simulink model "baxter_hybridcontroltraj2"  (Simulink 8.6)
settings: Solver=ode1  SolverMode=SingleTasking  StartTime=0.0  StopTime=stoptime  FixedStep=dt  RelTol=1e-3
values from neighbouring files (symbols this model uses):
  Aaug = [Ahat, zeros(14,7);Cpl(1:7,1:14), zeros(7)]    [mainMCVIntegralHybrid2_2d.m]
  Aaug1 = [Ahat1, zeros(14,7);Cpr(1:7,1:14), zeros(7)]    [mainMCVIntegralHybrid2_2d.m]
  Baug = [Bpl*Nbar Fhat; eye(7), zeros(7)]    [mainMCVIntegralHybrid2_2d.m]
  Baug1 = [Bpr*Nbar1 Fhat1; eye(7), zeros(7)]    [mainMCVIntegralHybrid2_2d.m]
  Caug = [eye(14),zeros(14,7)]    [mainMCVIntegralHybrid2_2d.m]
  Caug1 = [eye(14),zeros(14,7)]    [mainMCVIntegralHybrid2_2d.m]
  Daug = zeros(14,14)    [mainMCVIntegralHybrid2_2d.m]
  Daug1 = zeros(14,14)    [mainMCVIntegralHybrid2_2d.m]
  dt = 0.001    [mainMCVIntegralHybrid2_2d.m]
  faulttime = stoptime    (= 1795)    [mainMCVIntegralHybrid2_2d.m]
  initleft = [jlanglerow1(:,1)'+ 0.1*ones(1,7), zeros(1,14)]    [mainMCVIntegralHybrid2_2d.m]
  initright = [jranglerow1(:,1)'+ 0.1*ones(1,7),zeros(1,14)]    [mainMCVIntegralHybrid2_2d.m]
  Khat = Kplmcv    [mainMCVIntegralHybrid2_2d.m]
  seed = 0    [mainMCVIntegralHybrid2_2d.m]
  stepinput = [-0.36816     -0.55722      -1.1969       1.5731      0.99057       1.2609      0.60746].'    [mainMCVIntegralHybrid2_2d.m]
  stepinput1 = zeros(7,1)    [mainMCVIntegralHybrid2_2d.m]
  stepinput2 = [-0.36816     -0.55722      -1.1969       1.5731      0.99057       1.2609      0.60746].'    [mainMCVIntegralHybrid2_2d.m]
  steptime = 0.0    (= 0)    [mainMCVIntegralHybrid2_2d.m]
undefined symbols (not defined in the file or in its folder): jlanglerow, jranglerow, tanglerow
undefined symbols (not defined in the file): W
libraries: roblocks x14, powerlib_meascontrol x14
settings Model: Creator=Firdous  LastModifiedBy=Firdous
settings DataIOCC: LimitDataPoints=off  SaveFormat=Dataset  SignalLoggingSaveFormat=Dataset  ReturnWorkspaceOutputs=on
settings OptimizationCC: ExpressionDepthLimit=128
settings DebuggingCC: UnderspecifiedInitializationDetection=Simplified  MergeDetectMultiDrivingBlocksExec=error  SolverPrmCheckMsg=none  FcnCallInpInsideContextMsg=EnableAllAsError  AllowSymbolicDim=on  StateNameClashWarn=none  SFUnexpectedBacktrackingDiag=error  SFNoUnconditionalDefaultTransitionDiag=error
settings HardwareCC: ProdBitPerPointer=64  ProdLargestAtomicFloat=Float  ProdIntDivRoundTo=Zero  ProdEndianess=LittleEndian  ProdWordSize=64  ProdHWDeviceType=Intel->x86-64 (Windows64)
settings ModelReferenceCC: PropagateSignalLabelsOutOfModel=on
settings GRTTargetCC: TargetLangStandard=C99 (ISO)  GeneratePreprocessorConditionals=Use local settings  CombineOutputUpdateFcns=on  GRTInterface=off
settings ConfigComp: CovMetricSettings=dwe  CovHtmlReporting=off  CovSaveCumulativeToWorkspaceVar=off  CovSaveSingleToWorkspaceVar=off  CovExternalEMLEnable=on

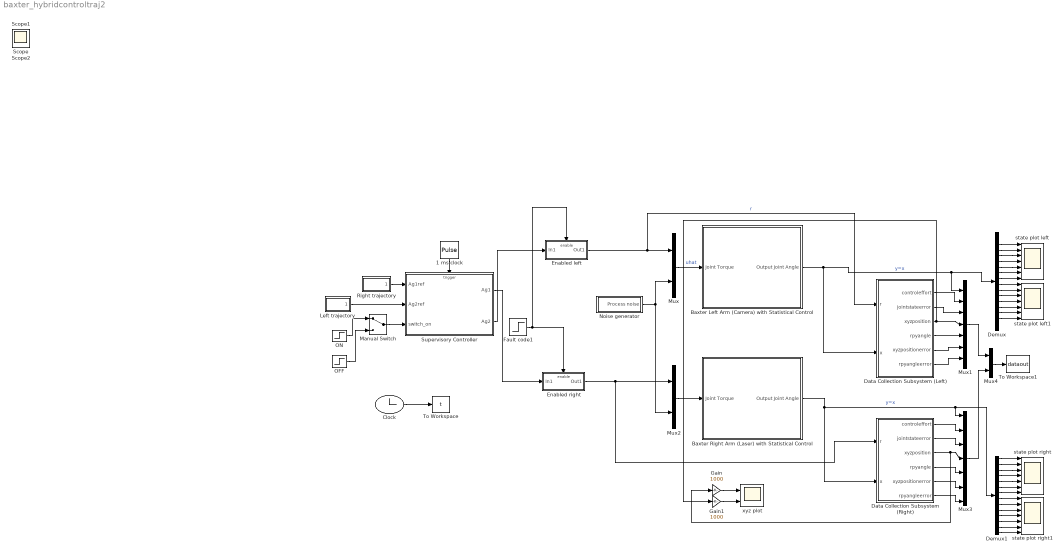
== system baxter_hybridcontroltraj2 ==
  1 ms clock : DiscretePulseGenerator  PulseType=Time based  Period=0.01  PulseWidth=10
  Baxter Left Arm (Camera) with Statistical Control : Subsystem
      mask Display: image('Baxter_Robot_from_RethinkRobotics_crop.jpg');
  Baxter Right Arm (Laser) with Statistical Control : Subsystem
      mask Display: image('Baxter_Robot_from_RethinkRobotics_crop.jpg');
  Clock : Clock
  Data Collection Subsystem (Left) : Subsystem
  Data Collection Subsystem (Right) : Subsystem
  Demux : Demux  Outputs=14
  Demux1 : Demux  Outputs=14
  Enabled left : Subsystem  TreatAsAtomicUnit=on
  Enabled right : Subsystem  TreatAsAtomicUnit=on
  Fault code1 : Step  Time=faulttime  Before=1  After=0  SampleTime=0
  Gain : Gain  Gain=1000
  Gain1 : Gain  Gain=1000
  Left trajectory : Subsystem
  Manual Switch : ManualSwitch
  Mux : Mux  Inputs=2
  Mux1 : Mux  Inputs=7
  Mux2 : Mux  Inputs=2
  Mux3 : Mux  Inputs=7
  Mux4 : Mux  Inputs=2
  Noise generator : Subsystem
  OFF : Step  Time=0  After=0  SampleTime=0
  ON : Step  Time=0  SampleTime=0
  Right trajectory : Subsystem
  Supervisory Controller : Stateflow chart  TreatAsAtomicUnit=on
  To Workspace : ToWorkspace  VariableName=t  SampleTime=-1
      settings: Decimation=10  Save2DSignal=2-D array (concatenate along first dimension)
  To Workspace1 : ToWorkspace  VariableName=dataout  SampleTime=-1
  state plot left : Scope  NumInputPorts=7
  state plot left1 : Scope  NumInputPorts=7
  state plot right : Scope  NumInputPorts=7
  state plot right1 : Scope  NumInputPorts=7
  xyz plot : Scope  NumInputPorts=2
  Scope : Scope
  Scope1 : Scope
  Scope2 : Scope
  wires:
  Baxter Left Arm (Camera) with Statistical Control/1(Output Joint Angle) -> Data Collection Subsystem (Left)/2(x), Demux/1, Mux1/1  "y=x"
  Enabled left/1(Out1) -> Data Collection Subsystem (Left)/1(r), Mux/1  "r"
  Clock/1 -> To Workspace/1
  Mux/1 -> Baxter Left Arm (Camera) with Statistical Control/1(Joint Torque)  "uhat"
  Data Collection Subsystem (Left)/1(controleffort) -> Mux1/2
  Data Collection Subsystem (Left)/2(jointstateerror) -> Mux1/3
  Data Collection Subsystem (Left)/3(xyzposition) -> Gain1/1, Mux1/4
  Data Collection Subsystem (Left)/4(rpyangle) -> Mux1/5
  Data Collection Subsystem (Left)/5(xyzpositionerror) -> Mux1/6
  Data Collection Subsystem (Left)/6(rpyangleerror) -> Mux1/7
  ON/1 -> Manual Switch/1
  OFF/1 -> Manual Switch/2
  Manual Switch/1 -> Supervisory Controller/3(switch_on)
  Mux2/1 -> Baxter Right Arm (Laser) with Statistical Control/1(Joint Torque)
  Enabled right/1(Out1) -> Data Collection Subsystem (Right)/1(r), Mux2/1
  Supervisory Controller/1(Ag1) -> Enabled right/1(In1)
  Supervisory Controller/2(Ag2) -> Enabled left/1(In1)
  Data Collection Subsystem (Right)/1(controleffort) -> Mux3/2
  Data Collection Subsystem (Right)/2(jointstateerror) -> Mux3/3
  Data Collection Subsystem (Right)/3(xyzposition) -> Gain/1, Mux3/4
  Data Collection Subsystem (Right)/4(rpyangle) -> Mux3/5
  Data Collection Subsystem (Right)/5(xyzpositionerror) -> Mux3/6
  Data Collection Subsystem (Right)/6(rpyangleerror) -> Mux3/7
  Mux4/1 -> To Workspace1/1
  Mux1/1 -> Mux4/1
  Mux3/1 -> Mux4/2
  Noise generator/1(Process noise) -> Mux2/2, Mux/2
  1 ms clock/1 -> Supervisory Controller/Trigger
  Fault code1/1 -> Enabled left/Enable, Enabled right/Enable
  Left trajectory/1(Left traj) -> Supervisory Controller/2(Ag2ref)
  Right trajectory/1(Right traj) -> Supervisory Controller/1(Ag1ref)
  Gain/1 -> xyz plot/1
  Gain1/1 -> xyz plot/2
  Demux/1 -> state plot left/1
  Demux/2 -> state plot left/2
  Demux/3 -> state plot left/3
  Demux/4 -> state plot left/4
  Demux/5 -> state plot left/5
  Demux/6 -> state plot left/6
  Demux/7 -> state plot left/7
  Baxter Right Arm (Laser) with Statistical Control/1(Output Joint Angle) -> Data Collection Subsystem (Right)/2(x), Demux1/1, Mux3/1  "y=x"
  Demux1/1 -> state plot right/1
  Demux1/2 -> state plot right/2
  Demux1/3 -> state plot right/3
  Demux1/4 -> state plot right/4
  Demux1/5 -> state plot right/5
  Demux1/6 -> state plot right/6
  Demux1/7 -> state plot right/7
  Demux/8 -> state plot left1/1
  Demux/9 -> state plot left1/2
  Demux/10 -> state plot left1/3
  Demux/11 -> state plot left1/4
  Demux/12 -> state plot left1/5
  Demux/13 -> state plot left1/6
  Demux/14 -> state plot left1/7
  Demux1/8 -> state plot right1/1
  Demux1/9 -> state plot right1/2
  Demux1/10 -> state plot right1/3
  Demux1/11 -> state plot right1/4
  Demux1/12 -> state plot right1/5
  Demux1/13 -> state plot right1/6
  Demux1/14 -> state plot right1/7

== system baxter_hybridcontroltraj2/Baxter Left Arm (Camera) with Statistical Control ==
  Joint Torque : Inport
  State-space model : StateSpace  A=Aaug  B=Baug  C=Caug  D=Daug  X0=initleft
  Output Joint Angle : Outport
  wires:
  State-space model/1 -> Output Joint Angle/1
  Joint Torque/1 -> State-space model/1

== system baxter_hybridcontroltraj2/Baxter Right Arm (Laser) with Statistical Control ==
  Joint Torque : Inport
  State-space model : StateSpace  A=Aaug1  B=Baug1  C=Caug1  D=Daug1  X0=initright
  Output Joint Angle : Outport
  wires:
  State-space model/1 -> Output Joint Angle/1
  Joint Torque/1 -> State-space model/1

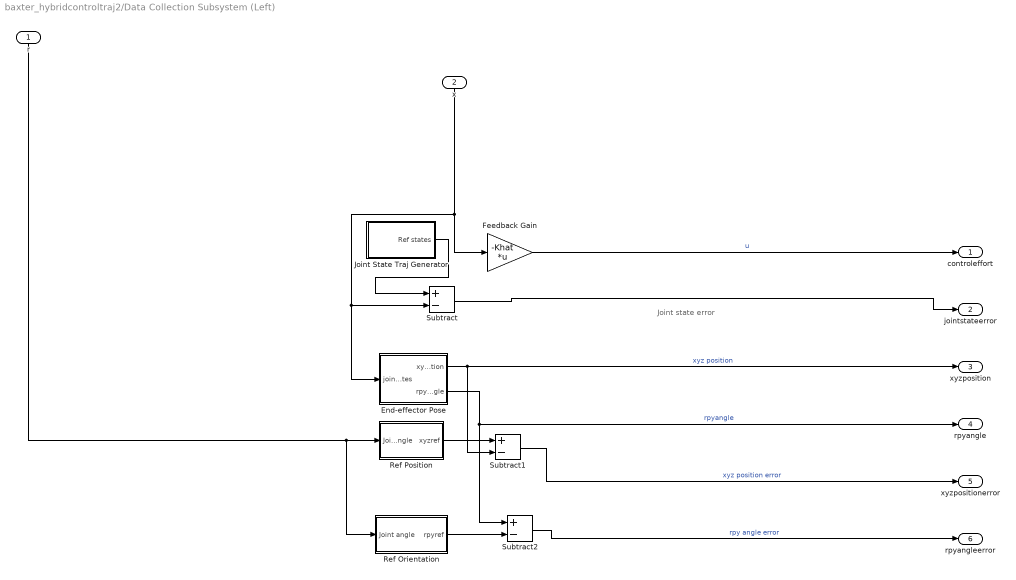
== system baxter_hybridcontroltraj2/Data Collection Subsystem (Left) ==
  note: Joint state error
  r : Inport
  x : Inport  Port=2
  End-effector Pose : Subsystem
  Feedback Gain : Gain  Gain=-Khat  Multiplication=Matrix(K*u)
  Joint State Traj Generator : Subsystem
  Ref Orientation : Subsystem
  Ref Position : Subsystem
  Subtract : Sum  Inputs=+-
  Subtract1 : Sum  Inputs=+-
  Subtract2 : Sum  Inputs=+-
  controleffort : Outport
  jointstateerror : Outport  Port=2
  xyzposition : Outport  Port=3
  rpyangle : Outport  Port=4
  xyzpositionerror : Outport  Port=5
  rpyangleerror : Outport  Port=6
  wires:
  Joint State Traj Generator/1(Ref states) -> Subtract/1
  Subtract/1 -> jointstateerror/1
  End-effector Pose/1(xyz Position) -> xyzposition/1, Subtract1/2  "xyz position"
  End-effector Pose/2(rpy Angle) -> rpyangle/1, Subtract2/1  "rpyangle"
  Ref Position/1(xyzref) -> Subtract1/1
  Subtract1/1 -> xyzpositionerror/1  "xyz position error"
  Feedback Gain/1 -> controleffort/1  "u"
  Ref Orientation/1(rpyref) -> Subtract2/2
  Subtract2/1 -> rpyangleerror/1  "rpy angle error"
  r/1 -> Ref Orientation/1(Joint angle), Ref Position/1(Joint angle)
  x/1 -> End-effector Pose/1(joint states), Subtract/2, Feedback Gain/1

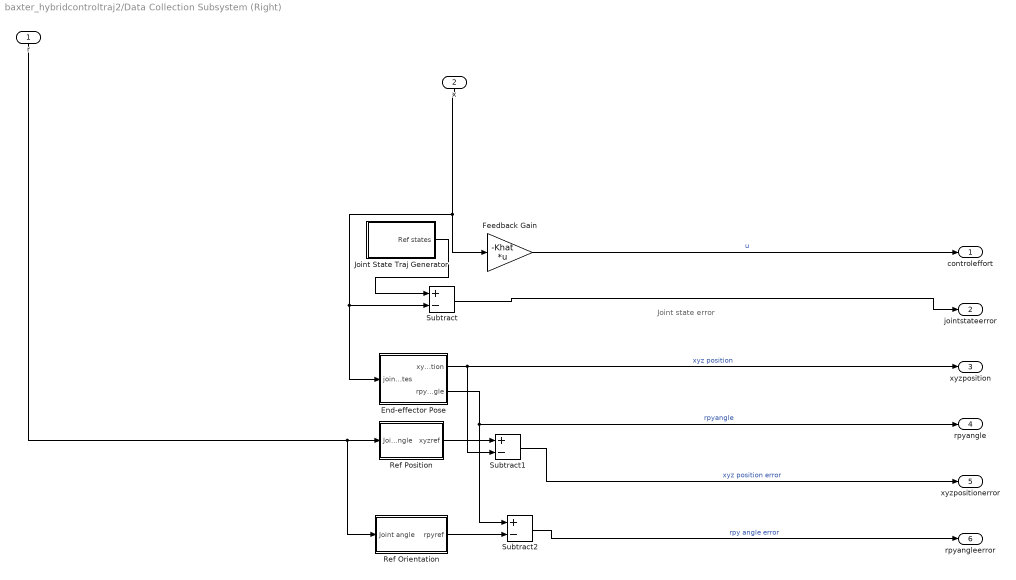
== system baxter_hybridcontroltraj2/Data Collection Subsystem (Right) ==
  note: Joint state error
  r : Inport
  x : Inport  Port=2
  End-effector Pose : Subsystem
  Feedback Gain : Gain  Gain=-Khat  Multiplication=Matrix(K*u)
  Joint State Traj Generator : Subsystem
  Ref Orientation : Subsystem
  Ref Position : Subsystem
  Subtract : Sum  Inputs=+-
  Subtract1 : Sum  Inputs=+-
  Subtract2 : Sum  Inputs=+-
  controleffort : Outport
  jointstateerror : Outport  Port=2
  xyzposition : Outport  Port=3
  rpyangle : Outport  Port=4
  xyzpositionerror : Outport  Port=5
  rpyangleerror : Outport  Port=6
  wires:
  Joint State Traj Generator/1(Ref states) -> Subtract/1
  Subtract/1 -> jointstateerror/1
  End-effector Pose/1(xyz Position) -> xyzposition/1, Subtract1/2  "xyz position"
  End-effector Pose/2(rpy Angle) -> rpyangle/1, Subtract2/1  "rpyangle"
  Ref Position/1(xyzref) -> Subtract1/1
  Subtract1/1 -> xyzpositionerror/1  "xyz position error"
  Feedback Gain/1 -> controleffort/1  "u"
  Ref Orientation/1(rpyref) -> Subtract2/2
  Subtract2/1 -> rpyangleerror/1  "rpy angle error"
  r/1 -> Ref Orientation/1(Joint angle), Ref Position/1(Joint angle)
  x/1 -> End-effector Pose/1(joint states), Subtract/2, Feedback Gain/1

== system baxter_hybridcontroltraj2/Enabled left ==
  In1 : Inport
  Enable : EnablePort
  Out1 : Outport
  wires:
  In1/1 -> Out1/1

== system baxter_hybridcontroltraj2/Enabled right ==
  In1 : Inport
  Enable : EnablePort
  Out1 : Outport
  wires:
  In1/1 -> Out1/1

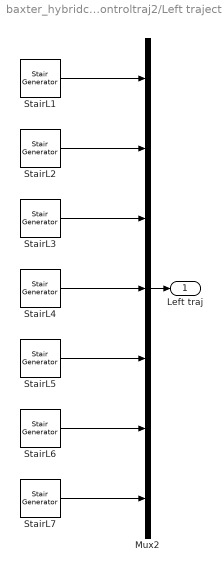
== system baxter_hybridcontroltraj2/Left trajectory ==
  Mux2 : Mux  Inputs=7
  StairL1 : powerlib_meascontrol/Pulse & Signal Generators/Stair Generator  t=tanglerow(1:15)  e=jlanglerow(1,:)  Ts=0
  StairL2 : powerlib_meascontrol/Pulse & Signal Generators/Stair Generator  t=tanglerow(1:15)  e=jlanglerow(2,:)  Ts=0
  StairL3 : powerlib_meascontrol/Pulse & Signal Generators/Stair Generator  t=tanglerow(1:15)  e=jlanglerow(3,:)  Ts=0
  StairL4 : powerlib_meascontrol/Pulse & Signal Generators/Stair Generator  t=tanglerow(1:15)  e=jlanglerow(4,:)  Ts=0
  StairL5 : powerlib_meascontrol/Pulse & Signal Generators/Stair Generator  t=tanglerow(1:15)  e=jlanglerow(5,:)  Ts=0
  StairL6 : powerlib_meascontrol/Pulse & Signal Generators/Stair Generator  t=tanglerow(1:15)  e=jlanglerow(6,:)  Ts=0
  StairL7 : powerlib_meascontrol/Pulse & Signal Generators/Stair Generator  t=tanglerow(1:15)  e=jlanglerow(7,:)  Ts=0
  Left traj : Outport
  wires:
  StairL2/1 -> Mux2/2
  StairL4/1 -> Mux2/4
  StairL7/1 -> Mux2/7
  StairL1/1 -> Mux2/1
  StairL3/1 -> Mux2/3
  StairL6/1 -> Mux2/6
  Mux2/1 -> Left traj/1
  StairL5/1 -> Mux2/5

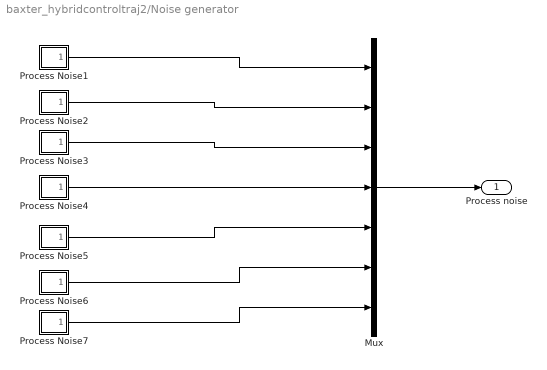
== system baxter_hybridcontroltraj2/Noise generator ==
  Mux : Mux  Inputs=7
  Process Noise1 : Subsystem  mask(Continuous White Noise.){Cov=W, Ts=dt, seed=seed}
      mask prompts: Cov "Noise Variance:"; Ts "Sample Time:"
      mask help:
      | White noise for continuous (s-domain) systems.
      | Band-limited using zero-order-hold.
      mask Help: Implemented using white noise into Zero Order Hold block. For faster simulation set sample time to highest value possible but in accordance with the fastest dynamics of system.
      mask Display: plot(1:20,rand(size(1:20)))
  Process Noise2 : Subsystem  mask(Continuous White Noise.){Cov=W, Ts=dt, seed=seed}
      mask prompts: Cov "Noise Variance:"; Ts "Sample Time:"
      mask help:
      | White noise for continuous (s-domain) systems.
      | Band-limited using zero-order-hold.
      mask Help: Implemented using white noise into Zero Order Hold block. For faster simulation set sample time to highest value possible but in accordance with the fastest dynamics of system.
      mask Display: plot(1:20,rand(size(1:20)))
  Process Noise3 : Subsystem  mask(Continuous White Noise.){Cov=W, Ts=dt, seed=seed}
      mask prompts: Cov "Noise Variance:"; Ts "Sample Time:"
      mask help:
      | White noise for continuous (s-domain) systems.
      | Band-limited using zero-order-hold.
      mask Help: Implemented using white noise into Zero Order Hold block. For faster simulation set sample time to highest value possible but in accordance with the fastest dynamics of system.
      mask Display: plot(1:20,rand(size(1:20)))
  Process Noise4 : Subsystem  mask(Continuous White Noise.){Cov=W, Ts=dt, seed=seed}
      mask prompts: Cov "Noise Variance:"; Ts "Sample Time:"
      mask help:
      | White noise for continuous (s-domain) systems.
      | Band-limited using zero-order-hold.
      mask Help: Implemented using white noise into Zero Order Hold block. For faster simulation set sample time to highest value possible but in accordance with the fastest dynamics of system.
      mask Display: plot(1:20,rand(size(1:20)))
  Process Noise5 : Subsystem  mask(Continuous White Noise.){Cov=W, Ts=dt, seed=seed}
      mask prompts: Cov "Noise Variance:"; Ts "Sample Time:"
      mask help:
      | White noise for continuous (s-domain) systems.
      | Band-limited using zero-order-hold.
      mask Help: Implemented using white noise into Zero Order Hold block. For faster simulation set sample time to highest value possible but in accordance with the fastest dynamics of system.
      mask Display: plot(1:20,rand(size(1:20)))
  Process Noise6 : Subsystem  mask(Continuous White Noise.){Cov=W, Ts=dt, seed=seed}
      mask prompts: Cov "Noise Variance:"; Ts "Sample Time:"
      mask help:
      | White noise for continuous (s-domain) systems.
      | Band-limited using zero-order-hold.
      mask Help: Implemented using white noise into Zero Order Hold block. For faster simulation set sample time to highest value possible but in accordance with the fastest dynamics of system.
      mask Display: plot(1:20,rand(size(1:20)))
  Process Noise7 : Subsystem  mask(Continuous White Noise.){Cov=W, Ts=dt, seed=seed}
      mask prompts: Cov "Noise Variance:"; Ts "Sample Time:"
      mask help:
      | White noise for continuous (s-domain) systems.
      | Band-limited using zero-order-hold.
      mask Help: Implemented using white noise into Zero Order Hold block. For faster simulation set sample time to highest value possible but in accordance with the fastest dynamics of system.
      mask Display: plot(1:20,rand(size(1:20)))
  Process noise : Outport
  wires:
  Process Noise2/1(out_1) -> Mux/2
  Process Noise1/1(out_1) -> Mux/1
  Process Noise3/1(out_1) -> Mux/3
  Process Noise4/1(out_1) -> Mux/4
  Process Noise5/1(out_1) -> Mux/5
  Process Noise6/1(out_1) -> Mux/6
  Process Noise7/1(out_1) -> Mux/7
  Mux/1 -> Process noise/1

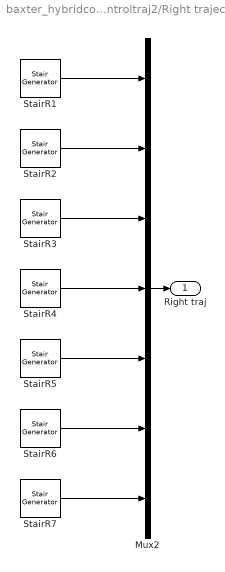
== system baxter_hybridcontroltraj2/Right trajectory ==
  Mux2 : Mux  Inputs=7
  StairR1 : powerlib_meascontrol/Pulse & Signal Generators/Stair Generator  t=tanglerow(1:15)  e=jranglerow(1,:)  Ts=0
  StairR2 : powerlib_meascontrol/Pulse & Signal Generators/Stair Generator  t=tanglerow(1:15)  e=jranglerow(2,:)  Ts=0
  StairR3 : powerlib_meascontrol/Pulse & Signal Generators/Stair Generator  t=tanglerow(1:15)  e=jranglerow(3,:)  Ts=0
  StairR4 : powerlib_meascontrol/Pulse & Signal Generators/Stair Generator  t=tanglerow(1:15)  e=jranglerow(4,:)  Ts=0
  StairR5 : powerlib_meascontrol/Pulse & Signal Generators/Stair Generator  t=tanglerow(1:15)  e=jranglerow(5,:)  Ts=0
  StairR6 : powerlib_meascontrol/Pulse & Signal Generators/Stair Generator  t=tanglerow(1:15)  e=jranglerow(6,:)  Ts=0
  StairR7 : powerlib_meascontrol/Pulse & Signal Generators/Stair Generator  t=tanglerow(1:15)  e=jranglerow(7,:)  Ts=0
  Right traj : Outport
  wires:
  StairR2/1 -> Mux2/2
  StairR4/1 -> Mux2/4
  StairR7/1 -> Mux2/7
  StairR1/1 -> Mux2/1
  StairR3/1 -> Mux2/3
  StairR6/1 -> Mux2/6
  Mux2/1 -> Right traj/1
  StairR5/1 -> Mux2/5

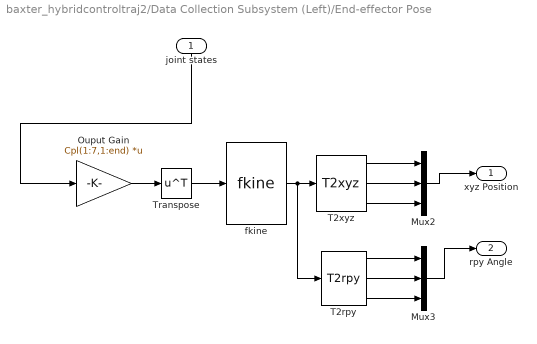
== system baxter_hybridcontroltraj2/Data Collection Subsystem (Left)/End-effector Pose ==
  joint states : Inport
  Mux2 : Mux  Inputs=3
  Mux3 : Mux  Inputs=3
  Ouput Gain : Gain  Gain=Cpl(1:7,1:end)  Multiplication=Matrix(K*u)
  T2rpy : roblocks/Transform Conversion/T2rpy
  T2xyz : roblocks/Transform Conversion/T2xyz
  Transpose : Math  Operator=transpose  SaturateOnIntegerOverflow=on
  fkine : roblocks/Kinematics/fkine  robot=left
  xyz Position : Outport
  rpy Angle : Outport  Port=2
  wires:
  fkine/1 -> T2rpy/1, T2xyz/1
  T2xyz/2 -> Mux2/2
  T2xyz/3 -> Mux2/3
  Mux2/1 -> xyz Position/1
  Ouput Gain/1 -> Transpose/1
  T2xyz/1 -> Mux2/1
  Transpose/1 -> fkine/1
  T2rpy/1 -> Mux3/1
  T2rpy/3 -> Mux3/3
  Mux3/1 -> rpy Angle/1
  T2rpy/2 -> Mux3/2
  joint states/1 -> Ouput Gain/1

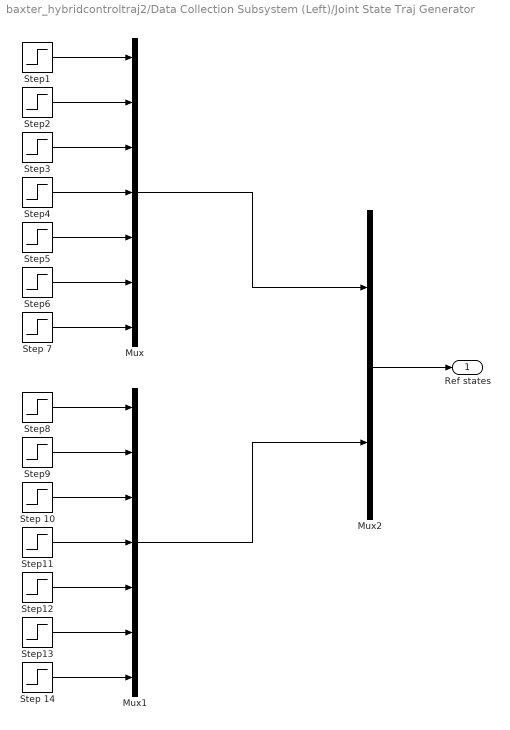
== system baxter_hybridcontroltraj2/Data Collection Subsystem (Left)/Joint State Traj Generator ==
  Mux : Mux  Inputs=7
  Mux1 : Mux  Inputs=7
  Mux2 : Mux  Inputs=2
  Step 10 : Step  Time=steptime  After=stepinput1(3)  SampleTime=0
  Step 14 : Step  Time=steptime  After=stepinput1(7)  SampleTime=0
  Step 7 : Step  Time=steptime  After=stepinput(7)  SampleTime=0
  Step1 : Step  Time=steptime  After=stepinput(1)  SampleTime=0
  Step11 : Step  Time=steptime  After=stepinput1(4)  SampleTime=0
  Step12 : Step  Time=steptime  After=stepinput1(5)  SampleTime=0
  Step13 : Step  Time=steptime  After=stepinput1(6)  SampleTime=0
  Step2 : Step  Time=steptime  After=stepinput(2)  SampleTime=0
  Step3 : Step  Time=steptime  After=stepinput(3)  SampleTime=0
  Step4 : Step  Time=steptime  After=stepinput(4)  SampleTime=0
  Step5 : Step  Time=steptime  After=stepinput(5)  SampleTime=0
  Step6 : Step  Time=steptime  After=stepinput(6)  SampleTime=0
  Step8 : Step  Time=steptime  After=stepinput1(1)  SampleTime=0
  Step9 : Step  Time=steptime  After=stepinput1(2)  SampleTime=0
  Ref states : Outport
  wires:
  Step1/1 -> Mux/1
  Step2/1 -> Mux/2
  Step3/1 -> Mux/3
  Step4/1 -> Mux/4
  Step5/1 -> Mux/5
  Step6/1 -> Mux/6
  Step 7/1 -> Mux/7
  Step8/1 -> Mux1/1
  Step9/1 -> Mux1/2
  Step 10/1 -> Mux1/3
  Step11/1 -> Mux1/4
  Step12/1 -> Mux1/5
  Step13/1 -> Mux1/6
  Step 14/1 -> Mux1/7
  Mux1/1 -> Mux2/2
  Mux/1 -> Mux2/1
  Mux2/1 -> Ref states/1

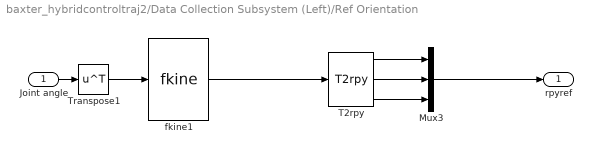
== system baxter_hybridcontroltraj2/Data Collection Subsystem (Left)/Ref Orientation ==
  Joint angle : Inport
  Mux3 : Mux  Inputs=3
  T2rpy : roblocks/Transform Conversion/T2rpy
  Transpose1 : Math  Operator=transpose  SaturateOnIntegerOverflow=on
  fkine1 : roblocks/Kinematics/fkine  robot=left
  rpyref : Outport
  wires:
  Joint angle/1 -> Transpose1/1
  Transpose1/1 -> fkine1/1
  fkine1/1 -> T2rpy/1
  T2rpy/3 -> Mux3/3
  Mux3/1 -> rpyref/1
  T2rpy/2 -> Mux3/2
  T2rpy/1 -> Mux3/1

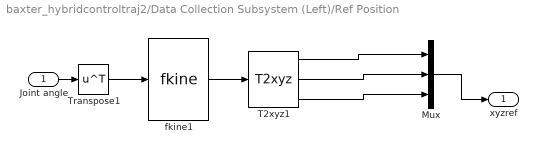
== system baxter_hybridcontroltraj2/Data Collection Subsystem (Left)/Ref Position ==
  Joint angle : Inport
  Mux : Mux  Inputs=3
  T2xyz1 : roblocks/Transform Conversion/T2xyz
  Transpose1 : Math  Operator=transpose  SaturateOnIntegerOverflow=on
  fkine1 : roblocks/Kinematics/fkine  robot=left
  xyzref : Outport
  wires:
  Joint angle/1 -> Transpose1/1
  Transpose1/1 -> fkine1/1
  fkine1/1 -> T2xyz1/1
  T2xyz1/3 -> Mux/3
  T2xyz1/1 -> Mux/1
  T2xyz1/2 -> Mux/2
  Mux/1 -> xyzref/1

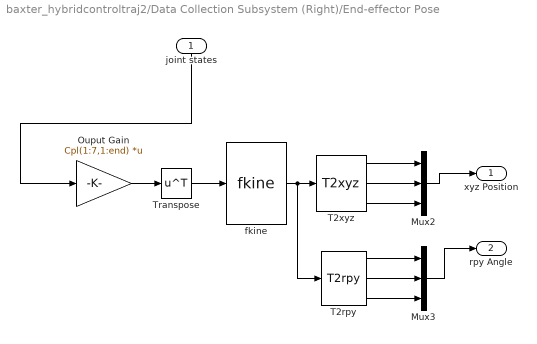
== system baxter_hybridcontroltraj2/Data Collection Subsystem (Right)/End-effector Pose ==
  joint states : Inport
  Mux2 : Mux  Inputs=3
  Mux3 : Mux  Inputs=3
  Ouput Gain : Gain  Gain=Cpl(1:7,1:end)  Multiplication=Matrix(K*u)
  T2rpy : roblocks/Transform Conversion/T2rpy
  T2xyz : roblocks/Transform Conversion/T2xyz
  Transpose : Math  Operator=transpose  SaturateOnIntegerOverflow=on
  fkine : roblocks/Kinematics/fkine  robot=right
  xyz Position : Outport
  rpy Angle : Outport  Port=2
  wires:
  fkine/1 -> T2rpy/1, T2xyz/1
  T2xyz/2 -> Mux2/2
  T2xyz/3 -> Mux2/3
  Mux2/1 -> xyz Position/1
  Ouput Gain/1 -> Transpose/1
  T2xyz/1 -> Mux2/1
  Transpose/1 -> fkine/1
  T2rpy/1 -> Mux3/1
  T2rpy/3 -> Mux3/3
  Mux3/1 -> rpy Angle/1
  T2rpy/2 -> Mux3/2
  joint states/1 -> Ouput Gain/1

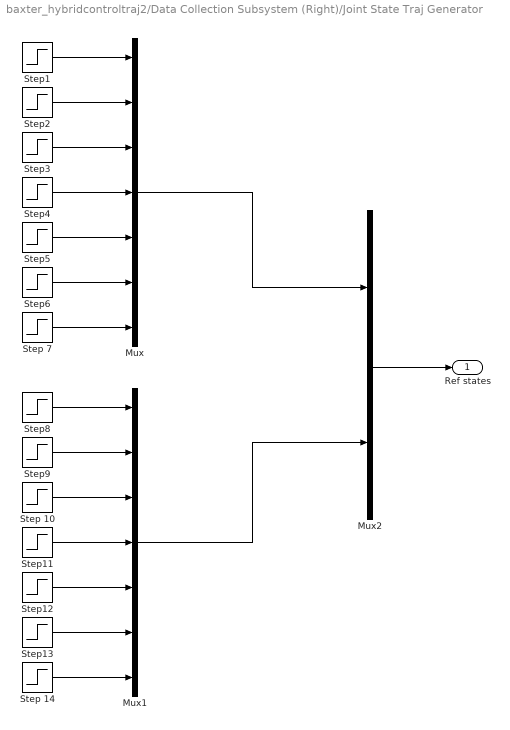
== system baxter_hybridcontroltraj2/Data Collection Subsystem (Right)/Joint State Traj Generator ==
  Mux : Mux  Inputs=7
  Mux1 : Mux  Inputs=7
  Mux2 : Mux  Inputs=2
  Step 10 : Step  Time=steptime  After=stepinput1(3)  SampleTime=0
  Step 14 : Step  Time=steptime  After=stepinput1(7)  SampleTime=0
  Step 7 : Step  Time=steptime  After=stepinput2(7)  SampleTime=0
  Step1 : Step  Time=steptime  After=stepinput2(1)  SampleTime=0
  Step11 : Step  Time=steptime  After=stepinput1(4)  SampleTime=0
  Step12 : Step  Time=steptime  After=stepinput1(5)  SampleTime=0
  Step13 : Step  Time=steptime  After=stepinput1(6)  SampleTime=0
  Step2 : Step  Time=steptime  After=stepinput2(2)  SampleTime=0
  Step3 : Step  Time=steptime  After=stepinput2(3)  SampleTime=0
  Step4 : Step  Time=steptime  After=stepinput2(4)  SampleTime=0
  Step5 : Step  Time=steptime  After=stepinput2(5)  SampleTime=0
  Step6 : Step  Time=steptime  After=stepinput2(6)  SampleTime=0
  Step8 : Step  Time=steptime  After=stepinput1(1)  SampleTime=0
  Step9 : Step  Time=steptime  After=stepinput1(2)  SampleTime=0
  Ref states : Outport
  wires:
  Step1/1 -> Mux/1
  Step2/1 -> Mux/2
  Step3/1 -> Mux/3
  Step4/1 -> Mux/4
  Step5/1 -> Mux/5
  Step6/1 -> Mux/6
  Step 7/1 -> Mux/7
  Step8/1 -> Mux1/1
  Step9/1 -> Mux1/2
  Step 10/1 -> Mux1/3
  Step11/1 -> Mux1/4
  Step12/1 -> Mux1/5
  Step13/1 -> Mux1/6
  Step 14/1 -> Mux1/7
  Mux1/1 -> Mux2/2
  Mux/1 -> Mux2/1
  Mux2/1 -> Ref states/1

== system baxter_hybridcontroltraj2/Data Collection Subsystem (Right)/Ref Orientation ==
  Joint angle : Inport
  Mux3 : Mux  Inputs=3
  T2rpy : roblocks/Transform Conversion/T2rpy
  Transpose1 : Math  Operator=transpose  SaturateOnIntegerOverflow=on
  fkine1 : roblocks/Kinematics/fkine  robot=right
  rpyref : Outport
  wires:
  Joint angle/1 -> Transpose1/1
  Transpose1/1 -> fkine1/1
  fkine1/1 -> T2rpy/1
  T2rpy/3 -> Mux3/3
  Mux3/1 -> rpyref/1
  T2rpy/2 -> Mux3/2
  T2rpy/1 -> Mux3/1

== system baxter_hybridcontroltraj2/Data Collection Subsystem (Right)/Ref Position ==
  Joint angle : Inport
  Mux : Mux  Inputs=3
  T2xyz1 : roblocks/Transform Conversion/T2xyz
  Transpose1 : Math  Operator=transpose  SaturateOnIntegerOverflow=on
  fkine1 : roblocks/Kinematics/fkine  robot=right
  xyzref : Outport
  wires:
  Joint angle/1 -> Transpose1/1
  Transpose1/1 -> fkine1/1
  fkine1/1 -> T2xyz1/1
  T2xyz1/3 -> Mux/3
  T2xyz1/1 -> Mux/1
  T2xyz1/2 -> Mux/2
  Mux/1 -> xyzref/1

== system baxter_hybridcontroltraj2/Noise generator/Process Noise1 ==
  White Noise : RandomNumber  Seed=seed  SampleTime=dt
  Zero Order Hold : DiscreteTransferFcn  Numerator=[sqrt(Cov)]  Denominator=[sqrt(Ts)]  SampleTime=Ts
  out_1 : Outport
  wires:
  Zero Order Hold/1 -> out_1/1
  White Noise/1 -> Zero Order Hold/1

== system baxter_hybridcontroltraj2/Noise generator/Process Noise2 ==
  White Noise : RandomNumber  Seed=seed  SampleTime=dt
  Zero Order Hold : DiscreteTransferFcn  Numerator=[sqrt(Cov)]  Denominator=[sqrt(Ts)]  SampleTime=Ts
  out_1 : Outport
  wires:
  Zero Order Hold/1 -> out_1/1
  White Noise/1 -> Zero Order Hold/1

== system baxter_hybridcontroltraj2/Noise generator/Process Noise3 ==
  White Noise : RandomNumber  Seed=seed  SampleTime=dt
  Zero Order Hold : DiscreteTransferFcn  Numerator=[sqrt(Cov)]  Denominator=[sqrt(Ts)]  SampleTime=Ts
  out_1 : Outport
  wires:
  Zero Order Hold/1 -> out_1/1
  White Noise/1 -> Zero Order Hold/1

== system baxter_hybridcontroltraj2/Noise generator/Process Noise4 ==
  White Noise : RandomNumber  Seed=seed  SampleTime=dt
  Zero Order Hold : DiscreteTransferFcn  Numerator=[sqrt(Cov)]  Denominator=[sqrt(Ts)]  SampleTime=Ts
  out_1 : Outport
  wires:
  Zero Order Hold/1 -> out_1/1
  White Noise/1 -> Zero Order Hold/1

== system baxter_hybridcontroltraj2/Noise generator/Process Noise5 ==
  White Noise : RandomNumber  Seed=seed  SampleTime=dt
  Zero Order Hold : DiscreteTransferFcn  Numerator=[sqrt(Cov)]  Denominator=[sqrt(Ts)]  SampleTime=Ts
  out_1 : Outport
  wires:
  Zero Order Hold/1 -> out_1/1
  White Noise/1 -> Zero Order Hold/1

== system baxter_hybridcontroltraj2/Noise generator/Process Noise6 ==
  White Noise : RandomNumber  Seed=seed  SampleTime=dt
  Zero Order Hold : DiscreteTransferFcn  Numerator=[sqrt(Cov)]  Denominator=[sqrt(Ts)]  SampleTime=Ts
  out_1 : Outport
  wires:
  Zero Order Hold/1 -> out_1/1
  White Noise/1 -> Zero Order Hold/1

== system baxter_hybridcontroltraj2/Noise generator/Process Noise7 ==
  White Noise : RandomNumber  Seed=seed  SampleTime=dt
  Zero Order Hold : DiscreteTransferFcn  Numerator=[sqrt(Cov)]  Denominator=[sqrt(Ts)]  SampleTime=Ts
  out_1 : Outport
  wires:
  Zero Order Hold/1 -> out_1/1
  White Noise/1 -> Zero Order Hold/1

== stateflow chart Supervisory Controller ==
  state Idle
  state Agent2Maneuver
    en:
    Ag2=Ag2ref;
  state Agent1Maneuver
    en:
    Ag1=Ag1ref;
  (default) -> Idle
  Idle -> Agent1Maneuver : [switch_on==1]
  Agent1Maneuver -> Idle [order 2] : [~switch_on==1]
  Agent1Maneuver -> Agent2Maneuver [order 1] : after(8,sec)
  Agent2Maneuver -> Agent1Maneuver : after(8,sec)
  data: Ag1 output double; Ag2 output double; Ag1ref input double; Ag2ref input double; switch_on input double
  events: call input RISING_EDGE_EVENT
